simulink model "F18_Linear_Model"  (R2018a)
settings: Solver=VariableStepAuto  StartTime=0.0  StopTime=600  RelTol=1e-3
PreLoadFcn:
  | F18_Linear
values from neighbouring files (symbols this model uses):
  A = [-0.0239, -28.316, 0, -32.2;      -0.0003, -0.3621, 1, 0;      0, -2.2115, -0.2532, 0;      0, 0, 1, 0]    [F18_Linear.m]
  B = [-3.8114, 0.00095;      -0.0515, 0;      -2.8791, 0;      0, 0]    [F18_Linear.m]
  C = diag([1,1,1,1])    [F18_Linear.m]
  C1 = [0 -1 0 1]    [F18_Linear.m]
  D = zeros(4,2)    [F18_Linear.m]
  d2r = pi/180    (= 0.0174532925199)    [F18_Linear.m]    (also in FA_18_Trim.m; FA_18_sfun.m; Sim.m)
  F1 = [-67.81 11973 -133.3 -11801]    [F18_Linear.m]
  F2 = 1414.2    [F18_Linear.m]
  Ini_cond = [438.6533;10*d2r;0*d2r;10*d2r]    [F18_Linear.m]
  Trimx_N = [365.74;15*d2r;0;15*d2r]    [F18_Linear.m]
settings Model: Creator=User  LastModifiedBy=User

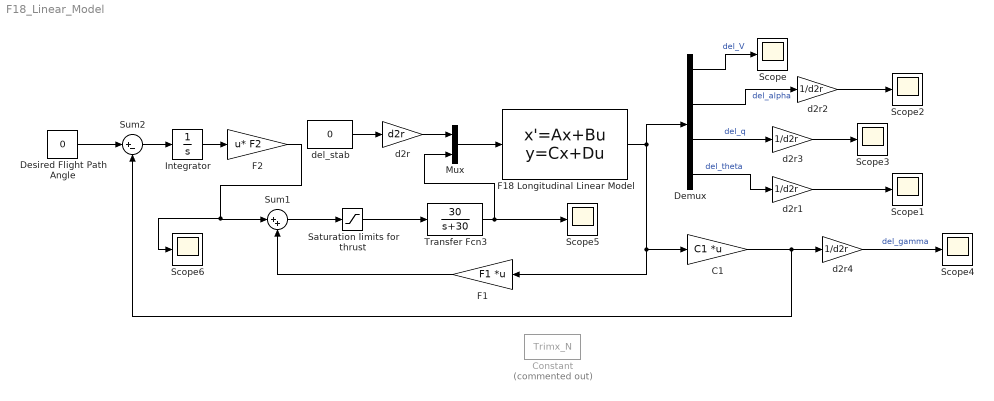
== system F18_Linear_Model ==
  C1 : Gain  Gain=C1  Multiplication=Matrix(K*u)
  Constant : Constant  Commented=on  Value=Trimx_N
  Demux : Demux
  Desired Flight Path Angle : Constant  Value=0
  F1 : Gain  Gain=F1  Multiplication=Matrix(K*u)
  F18 Longitudinal Linear Model : StateSpace  A=A  B=B  C=C  D=D  InitialCondition=Ini_cond
  F2 : Gain  Gain=F2  Multiplication=Matrix(u*K)
  Integrator : Integrator
  Mux : Mux  Inputs=2
  Saturation limits for thrust : Saturate  UpperLimit=20000  LowerLimit=0
  Scope{,1..6} (7 alike) : Scope
  Sum1 : Sum  Inputs=|++
  Sum2 : Sum  Inputs=|+-
  Transfer Fcn3 : TransferFcn  Numerator=[30]  Denominator=[1 30]
  d2r : Gain  Gain=d2r
  d2r{1..4} (4 alike) : Gain  Gain=1/d2r
  del_stab : Constant  Value=0
  wires:
  F18 Longitudinal Linear Model/1 -> F1/1, C1/1, Demux/1
  Sum2/1 -> Integrator/1
  Desired Flight Path Angle/1 -> Sum2/1
  C1/1 -> d2r4/1, Sum2/2
  Integrator/1 -> F2/1
  F2/1 -> Scope6/1, Sum1/1
  F1/1 -> Sum1/2
  Mux/1 -> F18 Longitudinal Linear Model/1
  del_stab/1 -> d2r/1
  d2r/1 -> Mux/1
  Demux/1 -> Scope/1  "del_V"
  Demux/4 -> d2r1/1  "del_theta"
  d2r1/1 -> Scope1/1
  d2r2/1 -> Scope2/1
  Demux/2 -> d2r2/1  "del_alpha"
  Demux/3 -> d2r3/1  "del_q"
  d2r3/1 -> Scope3/1
  Saturation limits for thrust/1 -> Transfer Fcn3/1
  Sum1/1 -> Saturation limits for thrust/1
  Transfer Fcn3/1 -> Mux/2, Scope5/1
  d2r4/1 -> Scope4/1  "del_gamma"
